simulink model "hybrid"  (R2022a)
settings: Solver=VariableStepAuto  StartTime=0.0  StopTime=T  RelTol=1e-3
values from neighbouring files (symbols this model uses):
  con = dss(A_c,[B1_c B2_c B3_c], [C1_c;C2_c], [D11_c, D12_c, D13_c; D21_c, D22_c, D23_c], eye(nx), config.parameters.time_delta)    [init_klmn.m]    (also in static_ozf.m = dss(A_c,[B1_c B2_c], [C1_c;C2_c], [D11_c, D12_c; D21_c, D22_)
  config = jsondecode(fileread(config_file_name))    [dh_analysis.m]    (also in init_klmn.m; static_ozf.m)
  lin_sys = dss(A_lin,[B_lin, A_lin], [C_lin; eye(nx)], [zeros(nzp,nwp), C_lin;zeros(ny,nwp), zeros(ny,nu)],eye(nx),config.parameters.time_delta)    [init_klmn.m]
  nu = nx    [dh_analysis.m]    (also in init_klmn.m; static_ozf.m)
  nwp = size(config.parameters.B_lin, 2)    [dh_analysis.m]    (also in init_klmn.m; static_ozf.m)
  nwu = 5    [basic_klmn.m]    (also in dh_analysis.m = config.parameters.nwu; init_klmn.m = config.parameters.nwu; static_ozf.m = config.parameters.nwu)
  nx = size(A,1)    [basic_klmn.m]    (also in dh_analysis.m = size(config.parameters.A_lin, 1); init_klmn.m = size(config.parameters.A_lin, 1); static_ozf.m = size(config.parameters.A_lin, 1))
  ny = nx    [basic_klmn.m]    (also in dh_analysis.m; init_klmn.m; static_ozf.m)
  nzp = size(config.parameters.C_lin, 1)    [dh_analysis.m]    (also in init_klmn.m; static_ozf.m)
  nzu = nwu    (= 5)    [basic_klmn.m]    (also in dh_analysis.m = nwu; init_klmn.m = nwu; static_ozf.m = nwu)
settings Model: Creator=jack  LastModifiedBy=jack

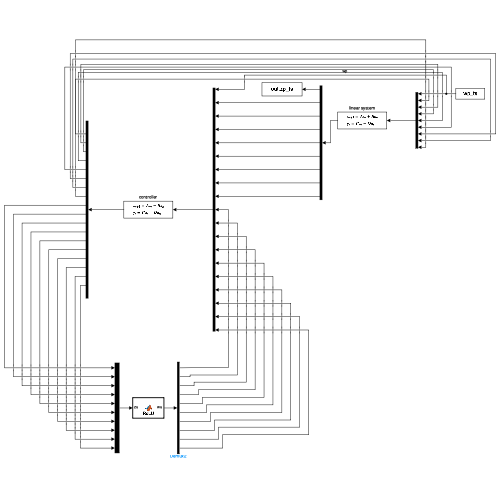
[thumbnail: Simulink's stored preview of the top-level diagram]
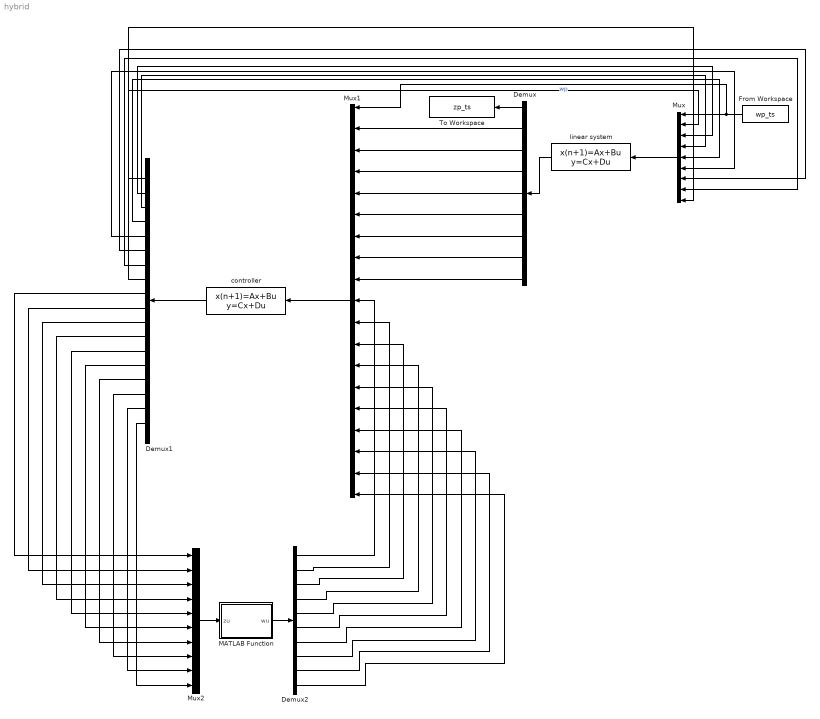
== system hybrid ==
  Demux : Demux  Outputs=nzp+ny
  Demux1 : Demux  Outputs=nu+nzu
  Demux2 : Demux  Outputs=nwu
  From Workspace : FromWorkspace  VariableName=wp_ts
  MATLAB Function : MATLAB Function  TreatAsAtomicUnit=on
  Mux : Mux  Inputs=nwp+nu
  Mux1 : Mux  Inputs=nwp+ny+nwu
  Mux2 : Mux  Inputs=nzu
  To Workspace : ToWorkspace  VariableName=zp_ts  SaveFormat=Timeseries  SampleTime=-1
  controller : DiscreteStateSpace  A=con.A  B=con.B  C=con.C  D=con.D  InitialCondition=zeros(nx,1)  SampleTime=config.parameters.time_delta
  linear system : DiscreteStateSpace  A=lin_sys.A  B=lin_sys.B  C=lin_sys.C  D=lin_sys.D  InitialCondition=zeros(nx,1)  SampleTime=config.parameters.time_delta
  wires:
  Mux/1 -> linear system/1
  From Workspace/1 -> Mux1/1, Mux/1  "wp"
  linear system/1 -> Demux/1
  Demux/1 -> To Workspace/1
  Demux/2 -> Mux1/2
  Demux/3 -> Mux1/3
  Demux/4 -> Mux1/4
  Demux/5 -> Mux1/5
  Demux/6 -> Mux1/6
  Demux/7 -> Mux1/7
  Demux/8 -> Mux1/8
  Demux/9 -> Mux1/9
  Mux1/1 -> controller/1
  controller/1 -> Demux1/1
  Demux1/1 -> Mux/2
  Demux1/2 -> Mux/3
  Demux1/3 -> Mux/4
  Demux1/4 -> Mux/5
  Demux1/5 -> Mux/6
  Demux1/6 -> Mux/7
  Demux1/7 -> Mux/8
  Demux1/8 -> Mux/9
  Demux1/9 -> Mux2/1
  Demux1/10 -> Mux2/2
  Demux1/11 -> Mux2/3
  Demux1/12 -> Mux2/4
  Demux1/13 -> Mux2/5
  Demux1/14 -> Mux2/6
  Demux1/15 -> Mux2/7
  Demux1/16 -> Mux2/8
  Demux1/17 -> Mux2/9
  Demux1/18 -> Mux2/10
  Mux2/1 -> MATLAB Function/1(zu)
  Demux2/1 -> Mux1/10
  Demux2/2 -> Mux1/11
  Demux2/3 -> Mux1/12
  Demux2/4 -> Mux1/13
  Demux2/5 -> Mux1/14
  Demux2/6 -> Mux1/15
  Demux2/7 -> Mux1/16
  Demux2/8 -> Mux1/17
  Demux2/9 -> Mux1/18
  Demux2/10 -> Mux1/19
  MATLAB Function/1(wu) -> Demux2/1

== matlab function hybrid/MATLAB Function ==
  data: zu input; wu output
function wu = ReLU(zu)

wu = max(zu,0);
